simulink model "Robot_Protected_Model"  (Simulink 8.0)
settings: Solver=ode45  StartTime=0.0  StopTime=simtime  RelTol=1e-3
values from neighbouring files (symbols this model uses):
  de = 30*pi/180    (= 0.523598775598)    [Robot_Feedback_Master.m]
  de0 = 0    [Robot_Feedback_Master.m]
  F = [mu1, 0; 0, mu2]    [Robot_Feedback_Master.m]
  g = 9.81    [Robot_Feedback_Master.m]
  Gamma1 = 0.0*diag([1, 1, 1, 1, 1, 1, 1, 1, 1], 0)    [Robot_Feedback_Master.m]
  I1 = 0.12    [Robot_Feedback_Master.m]
  Ie = 0.25    [Robot_Feedback_Master.m]
  Ie0 = 0.12    [Robot_Feedback_Master.m]
  initial_pos = 1*[-3; -3]    [Robot_Feedback_Master.m]
  initial_theta = 0*theta'    [Robot_Feedback_Master.m]
  initial_vel = 1*[-6; 6]    [Robot_Feedback_Master.m]
  KD = 100 * eye(2, 2)    [Robot_Feedback_Master.m]
  L1 = 1    [Robot_Feedback_Master.m]
  lambda = 0    [Robot_Feedback_Master.m]
  Lambda = 10 * eye(2, 2)    [Robot_Feedback_Master.m]
  lambdaf = 100    [Robot_Feedback_Master.m]
  Lc1 = 0.5    [Robot_Feedback_Master.m]
  Lce = 0.6    [Robot_Feedback_Master.m]
  Lce0 = 0.5    [Robot_Feedback_Master.m]
  M1 = 1    [Robot_Feedback_Master.m]
  Me = 5    [Robot_Feedback_Master.m]
  Me0 = 1    [Robot_Feedback_Master.m]
  R = 0 * eye(2, 2)    [Robot_Feedback_Master.m]
  tau1lim = 500    [Robot_Feedback_Master.m]
  tau2lim = 250    [Robot_Feedback_Master.m]
  thetaeps = 10    [Robot_Feedback_Master.m]
  thetamax = 40    [Robot_Feedback_Master.m]
undefined symbols (not defined in the file or in its folder): Gamma
libraries: dspmtrx3 x1
settings Model: Creator=Travis  LastModifiedBy=Dan
settings DataIOCC: SignalLoggingSaveFormat=ModelDataLogs
settings DebuggingCC: FcnCallInpInsideContextMsg=UseLocalSettings
settings GRTTargetCC: CombineOutputUpdateFcns=off  GRTInterface=on

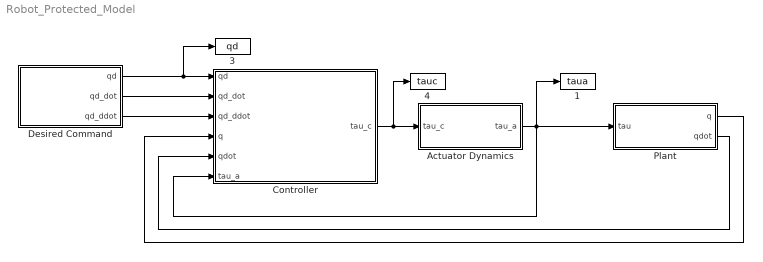
== system Robot_Protected_Model ==
  1 : ToWorkspace  VariableName=taua  SampleTime=-1  SaveFormat=Structure With Time
  3 : ToWorkspace  VariableName=qd  SampleTime=-1  SaveFormat=Structure With Time
  4 : ToWorkspace  VariableName=tauc  SampleTime=-1  SaveFormat=Structure With Time
  Actuator Dynamics : Subsystem
  Controller : Subsystem
  Desired Command : Subsystem
  Plant : Subsystem
  wires:
  Plant/2(qdot) -> Controller/5(qdot)
  Plant/1(q) -> Controller/4(q)
  Controller/1(tau_c) -> 4/1, Actuator Dynamics/1(tau_c)
  Desired Command/1(qd) -> Controller/1(qd), 3/1
  Actuator Dynamics/1(tau_a) -> Controller/6(tau_a), Plant/1(tau), 1/1
  Desired Command/2(qd_dot) -> Controller/2(qd_dot)
  Desired Command/3(qd_ddot) -> Controller/3(qd_ddot)

== system Robot_Protected_Model/Actuator Dynamics ==
  tau_c : Inport
  Demux : Demux  Outputs=2
  Mux : Mux  Inputs=2
  Saturation : Saturate  UpperLimit=tau1lim  LowerLimit=-tau1lim  ZeroCross=off
  Saturation1 : Saturate  UpperLimit=tau2lim  LowerLimit=-tau2lim  ZeroCross=off
  tau_a : Outport
  wires:
  Demux/1 -> Saturation/1
  Saturation/1 -> Mux/1
  Demux/2 -> Saturation1/1
  Saturation1/1 -> Mux/2
  Mux/1 -> tau_a/1
  tau_c/1 -> Demux/1

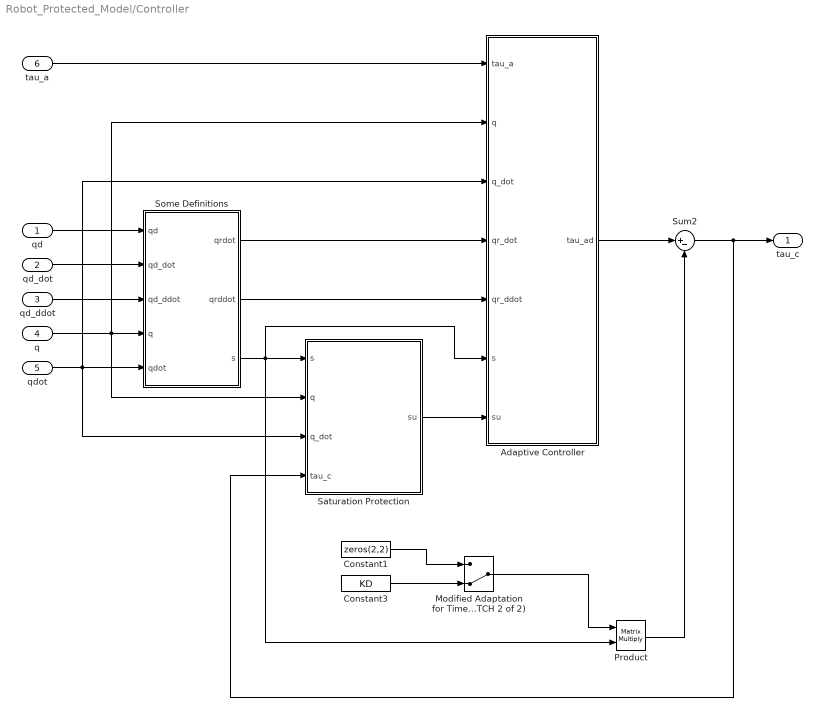
== system Robot_Protected_Model/Controller ==
  qd : Inport
  qd_dot : Inport  Port=2
  qd_ddot : Inport  Port=3
  q : Inport  Port=4
  qdot : Inport  Port=5
  tau_a : Inport  Port=6
  Adaptive Controller : Subsystem
  Constant1 : Constant  Value=zeros(2,2)
  Constant3 : Constant  Value=KD
  Modified Adaptation for Time Varying KD (SWITCH 2 of 2) : ManualSwitch  CurrentSetting=0
  Product : Product  Multiplication=Matrix(*)  RndMeth=Zero
  Saturation Protection : Subsystem
  Some Definitions : Subsystem
  Sum2 : Sum  Inputs=|+-
  tau_c : Outport
  wires:
  Adaptive Controller/1(tau_ad) -> Sum2/1
  Product/1 -> Sum2/2
  Sum2/1 -> tau_c/1, Saturation Protection/4(tau_c)
  q/1 -> Saturation Protection/2(q), Some Definitions/4(q), Adaptive Controller/2(q)
  qdot/1 -> Adaptive Controller/3(q_dot), Saturation Protection/3(q_dot), Some Definitions/5(qdot)
  Some Definitions/1(qrdot) -> Adaptive Controller/4(qr_dot)
  Some Definitions/2(qrddot) -> Adaptive Controller/5(qr_ddot)
  qd_ddot/1 -> Some Definitions/3(qd_ddot)
  qd_dot/1 -> Some Definitions/2(qd_dot)
  qd/1 -> Some Definitions/1(qd)
  Saturation Protection/1(su) -> Adaptive Controller/7(su)
  Some Definitions/3(s) -> Product/2, Adaptive Controller/6(s), Saturation Protection/1(s)
  Constant3/1 -> Modified Adaptation for Time Varying KD (SWITCH 2 of 2)/2
  Constant1/1 -> Modified Adaptation for Time Varying KD (SWITCH 2 of 2)/1
  Modified Adaptation for Time Varying KD (SWITCH 2 of 2)/1 -> Product/1
  tau_a/1 -> Adaptive Controller/1(tau_a)

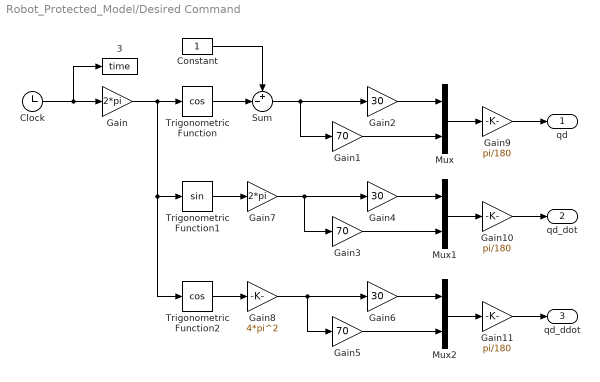
== system Robot_Protected_Model/Desired Command ==
  3 : ToWorkspace  VariableName=time  SampleTime=-1
  Clock : Clock
  Constant : Constant
  Gain : Gain  Gain=2*pi
  Gain1 : Gain  Gain=70
  Gain10 : Gain  Gain=pi/180
  Gain11 : Gain  Gain=pi/180
  Gain2 : Gain  Gain=30
  Gain3 : Gain  Gain=70
  Gain4 : Gain  Gain=30
  Gain5 : Gain  Gain=70
  Gain6 : Gain  Gain=30
  Gain7 : Gain  Gain=2*pi
  Gain8 : Gain  Gain=4*pi^2
  Gain9 : Gain  Gain=pi/180
  Mux : Mux  Inputs=2
  Mux1 : Mux  Inputs=2
  Mux2 : Mux  Inputs=2
  Sum : Sum  Inputs=+-|
  Trigonometric Function : Trigonometry  Operator=cos
  Trigonometric Function1 : Trigonometry
  Trigonometric Function2 : Trigonometry  Operator=cos
  qd : Outport
  qd_dot : Outport  Port=2
  qd_ddot : Outport  Port=3
  wires:
  Clock/1 -> Gain/1, 3/1
  Gain/1 -> Trigonometric Function/1, Trigonometric Function1/1, Trigonometric Function2/1
  Sum/1 -> Gain2/1, Gain1/1
  Gain1/1 -> Mux/2
  Trigonometric Function1/1 -> Gain7/1
  Trigonometric Function2/1 -> Gain8/1
  Mux/1 -> Gain9/1
  Gain2/1 -> Mux/1
  Gain7/1 -> Gain4/1, Gain3/1
  Gain3/1 -> Mux1/2
  Gain4/1 -> Mux1/1
  Gain8/1 -> Gain5/1, Gain6/1
  Gain5/1 -> Mux2/2
  Mux2/1 -> Gain11/1
  Gain6/1 -> Mux2/1
  Mux1/1 -> Gain10/1
  Constant/1 -> Sum/1
  Trigonometric Function/1 -> Sum/2
  Gain9/1 -> qd/1
  Gain10/1 -> qd_dot/1
  Gain11/1 -> qd_ddot/1

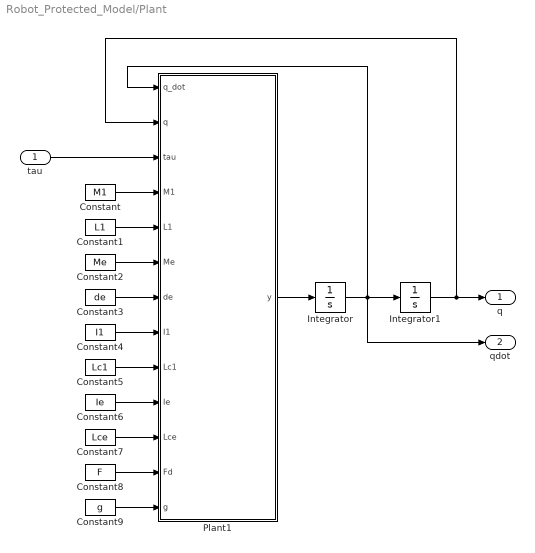
== system Robot_Protected_Model/Plant ==
  tau : Inport
  Constant : Constant  Value=M1
  Constant1 : Constant  Value=L1
  Constant2 : Constant  Value=Me
  Constant3 : Constant  Value=de
  Constant4 : Constant  Value=I1
  Constant5 : Constant  Value=Lc1
  Constant6 : Constant  Value=Ie
  Constant7 : Constant  Value=Lce
  Constant8 : Constant  Value=F
  Constant9 : Constant  Value=g
  Integrator : Integrator  InitialCondition=initial_vel
  Integrator1 : Integrator  InitialCondition=initial_pos
  Plant1 : MATLAB Function  TreatAsAtomicUnit=on
  q : Outport
  qdot : Outport  Port=2
  wires:
  Plant1/1(y) -> Integrator/1
  Integrator/1 -> qdot/1, Plant1/1(q_dot), Integrator1/1
  Constant/1 -> Plant1/4(M1)
  Constant1/1 -> Plant1/5(L1)
  Constant2/1 -> Plant1/6(Me)
  Constant3/1 -> Plant1/7(de)
  Constant5/1 -> Plant1/9(Lc1)
  Constant4/1 -> Plant1/8(I1)
  Constant6/1 -> Plant1/10(Ie)
  Constant7/1 -> Plant1/11(Lce)
  tau/1 -> Plant1/3(tau)
  Integrator1/1 -> Plant1/2(q), q/1
  Constant8/1 -> Plant1/12(Fd)
  Constant9/1 -> Plant1/13(g)

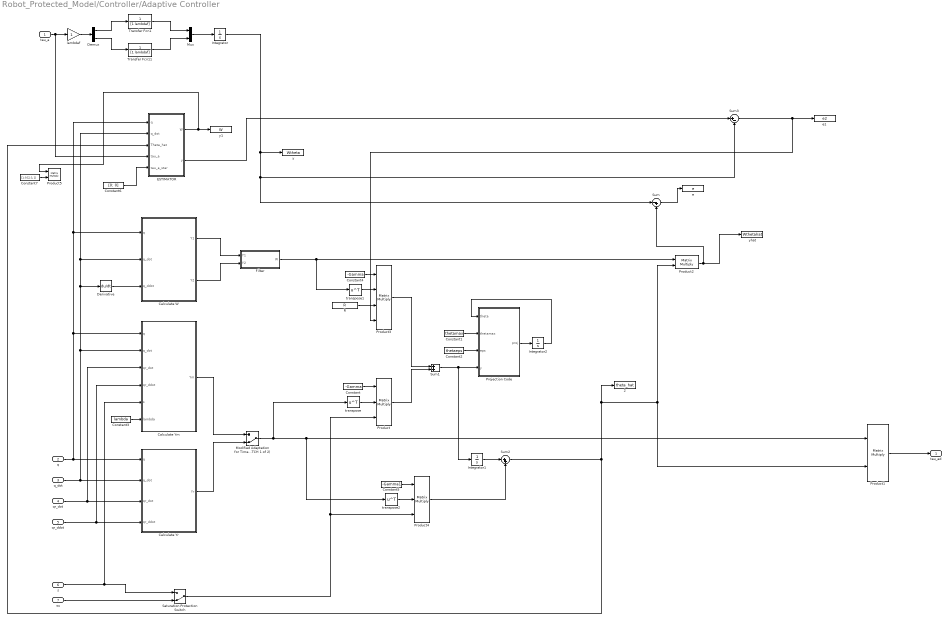
== system Robot_Protected_Model/Controller/Adaptive Controller ==
  tau_a : Inport
  q : Inport  Port=2
  q_dot : Inport  Port=3
  qr_dot : Inport  Port=4
  qr_ddot : Inport  Port=5
  s : Inport  Port=6
  su : Inport  Port=7
  2 : ToWorkspace  VariableName=theta_hat  SampleTime=-1  SaveFormat=Structure With Time
  Calculate W : MATLAB Function  TreatAsAtomicUnit=on
  Calculate Ym : MATLAB Function  TreatAsAtomicUnit=on
  Calculate Yr : MATLAB Function  TreatAsAtomicUnit=on
  Constant : Constant  Value=-Gamma
  Constant1 : Constant  Value=thetamax
  Constant2 : Constant  Value=thetaeps
  Constant3 : Constant  Value=lambda
  Constant4 : Constant  Value=-Gamma
  Constant5 : Constant  Value=-Gamma1
  Constant6 : Constant  Value=[0; 0]
  Constant7 : Constant  Value=[1; 0.12; 1; 1]
  Demux : Demux  Outputs=2
  Derivative : Derivative
  ESTIMATOR : Subsystem
  Filter : Subsystem
  Integrator : Integrator  InitialCondition=[0; 0]
  Integrator1 : Integrator  InitialCondition=initial_theta
  Integrator2 : Integrator  InitialCondition=initial_theta
  Modified Adaptation for Time Varying KD (SWITCH 1 of 2) : ManualSwitch  CurrentSetting=0
  Mux : Mux  Inputs=2
  Product : Product  Inputs=3  Multiplication=Matrix(*)  RndMeth=Zero
  Product1 : Product  Multiplication=Matrix(*)  RndMeth=Zero
  Product2 : Product  Multiplication=Matrix(*)  RndMeth=Zero
  Product3 : Product  Inputs=4  Multiplication=Matrix(*)  RndMeth=Zero
  Product4 : Product  Inputs=3  Multiplication=Matrix(*)  RndMeth=Zero
  Product5 : Product  Multiplication=Matrix(*)  RndMeth=Zero
  Projection Code : Subsystem
  R : Constant  Value=R
  Saturation Protection Switch : ManualSwitch  CurrentSetting=0
  Sum : Sum  Inputs=|-+
  Sum1 : Sum
  Sum2 : Sum  Inputs=|++
  Sum3 : Sum  Inputs=|+-
  Transfer Fcn1 : TransferFcn  Denominator=[1 lambdaf]
  Transfer Fcn11 : TransferFcn  Denominator=[1 lambdaf]
  e : ToWorkspace  VariableName=e  SampleTime=-1  SaveFormat=Structure With Time
  e1 : ToWorkspace  VariableName=e2  SampleTime=-1  SaveFormat=Structure With Time
  lambdaf : Gain
  transpose : Math  Operator=transpose  SaturateOnIntegerOverflow=on
  transpose1 : Math  Operator=transpose  SaturateOnIntegerOverflow=on
  transpose2 : Math  Operator=transpose  SaturateOnIntegerOverflow=on
  y : ToWorkspace  VariableName=Wtheta  SampleTime=-1  SaveFormat=Structure With Time
  y1 : ToWorkspace  VariableName=W  SampleTime=-1  SaveFormat=Structure With Time
  yhat : ToWorkspace  VariableName=Wthetahat  SampleTime=-1  SaveFormat=Structure With Time
  tau_ad : Outport
  wires:
  Constant/1 -> Product/1
  transpose/1 -> Product/2
  Product1/1 -> tau_ad/1
  q/1 -> Calculate Yr/1(q), Calculate Ym/1(q), ESTIMATOR/1(q), Calculate W/1(q)
  qr_ddot/1 -> Calculate Ym/4(qr_ddot), Calculate Yr/4(qr_ddot)
  qr_dot/1 -> Calculate Ym/3(qr_dot), Calculate Yr/3(qr_dot)
  q_dot/1 -> Derivative/1, ESTIMATOR/2(q_dot), Calculate W/2(q_dot), Calculate Ym/2(q_dot), Calculate Yr/2(q_dot)
  s/1 -> Calculate Ym/5(s), Saturation Protection Switch/1
  su/1 -> Saturation Protection Switch/2
  Saturation Protection Switch/1 -> Product4/3, Product/3
  Constant3/1 -> Calculate Ym/6(lambda)
  Modified Adaptation for Time Varying KD (SWITCH 1 of 2)/1 -> transpose/1, transpose2/1, Product1/1
  Calculate Ym/1(Ym) -> Modified Adaptation for Time Varying KD (SWITCH 1 of 2)/1
  Calculate Yr/1(Yr) -> Modified Adaptation for Time Varying KD (SWITCH 1 of 2)/2
  Derivative/1 -> Calculate W/3(q_ddot)
  Calculate W/1(Y1) -> Filter/1(Y1)
  Calculate W/2(Y2) -> Filter/2(Y2)
  Demux/1 -> Transfer Fcn1/1
  Demux/2 -> Transfer Fcn11/1
  tau_a/1 -> ESTIMATOR/4(tau_a), lambdaf/1
  Transfer Fcn1/1 -> Mux/1
  Transfer Fcn11/1 -> Mux/2
  Mux/1 -> Integrator/1
  Filter/1(W) -> transpose1/1, Product2/1
  Integrator/1 -> Sum3/2, Sum/1, y/1
  Product2/1 -> yhat/1, Sum/2
  Sum/1 -> e/1
  Projection Code/1(proj) -> Integrator2/1
  Constant1/1 -> Projection Code/2(thetamax)
  Constant2/1 -> Projection Code/3(eps)
  Sum2/1 -> 2/1, Product1/2, Product2/2, ESTIMATOR/3(Theta_hat)
  Constant4/1 -> Product3/1
  transpose1/1 -> Product3/2
  R/1 -> Product3/3
  Product3/1 -> Sum1/1
  Product/1 -> Sum1/2
  Sum1/1 -> Integrator1/1, Projection Code/4(y)
  lambdaf/1 -> Demux/1
  Integrator2/1 -> Projection Code/1(theta)
  Constant5/1 -> Product4/1
  transpose2/1 -> Product4/2
  Product4/1 -> Sum2/2
  ESTIMATOR/1(W) -> Product5/1, y1/1
  Integrator1/1 -> Sum2/1
  Constant7/1 -> Product5/2
  ESTIMATOR/2(y) -> Sum3/1
  Sum3/1 -> Product3/4, e1/1
  Constant6/1 -> ESTIMATOR/5(tau_a_star)

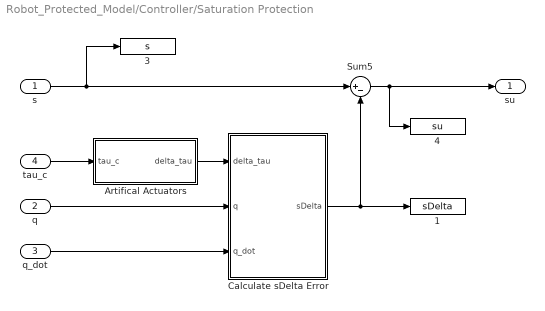
== system Robot_Protected_Model/Controller/Saturation Protection ==
  s : Inport
  q : Inport  Port=2
  q_dot : Inport  Port=3
  tau_c : Inport  Port=4
  1 : ToWorkspace  VariableName=sDelta  SampleTime=-1  SaveFormat=Structure With Time
  3 : ToWorkspace  VariableName=s  SampleTime=-1  SaveFormat=Structure With Time
  4 : ToWorkspace  VariableName=su  SampleTime=-1  SaveFormat=Structure With Time
  Artifical Actuators : Subsystem
  "Calculate sDelta Error " : Subsystem
  Sum5 : Sum  Inputs=|+-
  su : Outport
  wires:
  q/1 -> "Calculate sDelta Error "/2(q)
  q_dot/1 -> "Calculate sDelta Error "/3(q_dot)
  Artifical Actuators/1(delta_tau) -> "Calculate sDelta Error "/1(delta_tau)
  s/1 -> 3/1, Sum5/1
  Sum5/1 -> su/1, 4/1
  "Calculate sDelta Error "/1(sDelta) -> 1/1, Sum5/2
  tau_c/1 -> Artifical Actuators/1(tau_c)

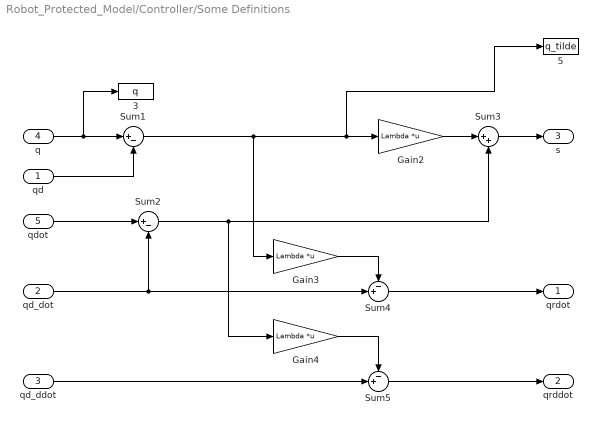
== system Robot_Protected_Model/Controller/Some Definitions ==
  qd : Inport
  qd_dot : Inport  Port=2
  qd_ddot : Inport  Port=3
  q : Inport  Port=4
  qdot : Inport  Port=5
  3 : ToWorkspace  VariableName=q  SampleTime=-1  SaveFormat=Structure With Time
  5 : ToWorkspace  VariableName=q_tilde  SampleTime=-1  SaveFormat=Structure With Time
  Gain2 : Gain  Gain=Lambda  Multiplication=Matrix(K*u)
  Gain3 : Gain  Gain=Lambda  Multiplication=Matrix(K*u)
  Gain4 : Gain  Gain=Lambda  Multiplication=Matrix(K*u)
  Sum1 : Sum  Inputs=|+-
  Sum2 : Sum  Inputs=|+-
  Sum3 : Sum  Inputs=|++
  Sum4 : Sum  Inputs=-+|
  Sum5 : Sum  Inputs=-+|
  qrdot : Outport
  qrddot : Outport  Port=2
  s : Outport  Port=3
  wires:
  qd/1 -> Sum1/2
  qd_dot/1 -> Sum2/2, Sum4/2
  q/1 -> 3/1, Sum1/1
  Sum1/1 -> Gain3/1, 5/1, Gain2/1
  qdot/1 -> Sum2/1
  Sum2/1 -> Sum3/2, Gain4/1
  Gain2/1 -> Sum3/1
  Sum3/1 -> s/1
  Sum4/1 -> qrdot/1
  Sum5/1 -> qrddot/1
  Gain3/1 -> Sum4/1
  Gain4/1 -> Sum5/1
  qd_ddot/1 -> Sum5/2

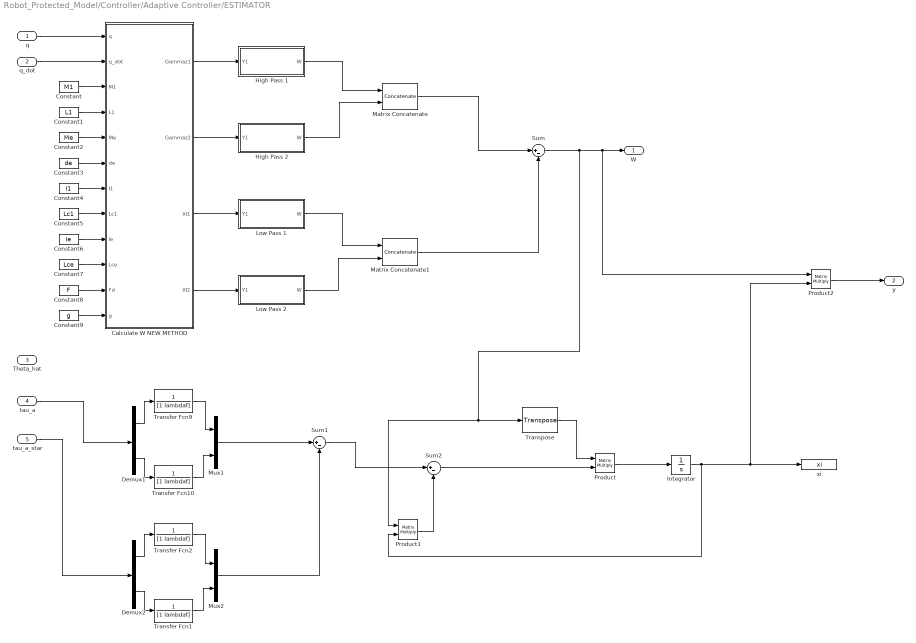
== system Robot_Protected_Model/Controller/Adaptive Controller/ESTIMATOR ==
  q : Inport
  q_dot : Inport  Port=2
  Theta_hat : Inport  Port=3
  tau_a : Inport  Port=4
  tau_a_star : Inport  Port=5
  Calculate W NEW METHOD : MATLAB Function  TreatAsAtomicUnit=on
  Constant : Constant  Value=M1
  Constant1 : Constant  Value=L1
  Constant2 : Constant  Value=Me
  Constant3 : Constant  Value=de
  Constant4 : Constant  Value=I1
  Constant5 : Constant  Value=Lc1
  Constant6 : Constant  Value=Ie
  Constant7 : Constant  Value=Lce
  Constant8 : Constant  Value=F
  Constant9 : Constant  Value=g
  Demux1 : Demux  Outputs=2
  Demux2 : Demux  Outputs=2
  High Pass 1 : Subsystem
  High Pass 2 : Subsystem
  Integrator : Integrator  InitialCondition=[0; 0; 0; 0]
  Low Pass 1 : Subsystem
  Low Pass 2 : Subsystem
  Matrix Concatenate : Concatenate  Mode=Multidimensional array
  Matrix Concatenate1 : Concatenate  Mode=Multidimensional array
  Mux1 : Mux  Inputs=2
  Mux2 : Mux  Inputs=2
  Product : Product  Multiplication=Matrix(*)  RndMeth=Zero
  Product1 : Product  Multiplication=Matrix(*)  RndMeth=Zero
  Product2 : Product  Multiplication=Matrix(*)  RndMeth=Zero
  Sum : Sum  Inputs=|+-
  Sum1 : Sum  Inputs=|+-
  Sum2 : Sum  Inputs=|+-
  Transfer Fcn{1..2,9..10} (4 alike) : TransferFcn  Denominator=[1 lambdaf]
  Transpose : dspmtrx3/Transpose  Hermitian=off  overflowFlag=off
  xi : ToWorkspace  VariableName=xi  SampleTime=-1  SaveFormat=Structure With Time
  W : Outport
  y : Outport  Port=2
  wires:
  Constant/1 -> Calculate W NEW METHOD/3(M1)
  Constant1/1 -> Calculate W NEW METHOD/4(L1)
  Constant2/1 -> Calculate W NEW METHOD/5(Me)
  Constant3/1 -> Calculate W NEW METHOD/6(de)
  Constant4/1 -> Calculate W NEW METHOD/7(I1)
  Constant5/1 -> Calculate W NEW METHOD/8(Lc1)
  Constant6/1 -> Calculate W NEW METHOD/9(Ie)
  Constant7/1 -> Calculate W NEW METHOD/10(Lce)
  Constant8/1 -> Calculate W NEW METHOD/11(Fd)
  Constant9/1 -> Calculate W NEW METHOD/12(g)
  q/1 -> Calculate W NEW METHOD/1(q)
  q_dot/1 -> Calculate W NEW METHOD/2(q_dot)
  Calculate W NEW METHOD/3(XI1) -> Low Pass 1/1(Y1)
  Calculate W NEW METHOD/4(XI2) -> Low Pass 2/1(Y1)
  Calculate W NEW METHOD/2(Gammaz2) -> High Pass 2/1(Y1)
  Calculate W NEW METHOD/1(Gammaz1) -> High Pass 1/1(Y1)
  High Pass 1/1(W) -> Matrix Concatenate/1
  High Pass 2/1(W) -> Matrix Concatenate/2
  Low Pass 1/1(W) -> Matrix Concatenate1/1
  Low Pass 2/1(W) -> Matrix Concatenate1/2
  Matrix Concatenate/1 -> Sum/1
  Matrix Concatenate1/1 -> Sum/2
  Sum/1 -> Product1/1, Transpose/1, Product2/1, W/1
  Demux1/1 -> Transfer Fcn9/1
  Transfer Fcn9/1 -> Mux1/1
  Demux1/2 -> Transfer Fcn10/1
  Transfer Fcn10/1 -> Mux1/2
  Demux2/1 -> Transfer Fcn2/1
  Transfer Fcn2/1 -> Mux2/1
  Demux2/2 -> Transfer Fcn1/1
  Transfer Fcn1/1 -> Mux2/2
  tau_a/1 -> Demux1/1
  tau_a_star/1 -> Demux2/1
  Mux1/1 -> Sum1/1
  Mux2/1 -> Sum1/2
  Transpose/1 -> Product/1
  Sum2/1 -> Product/2
  Product/1 -> Integrator/1
  Sum1/1 -> Sum2/1
  Product1/1 -> Sum2/2
  Integrator/1 -> Product1/2, Product2/2, xi/1
  Product2/1 -> y/1

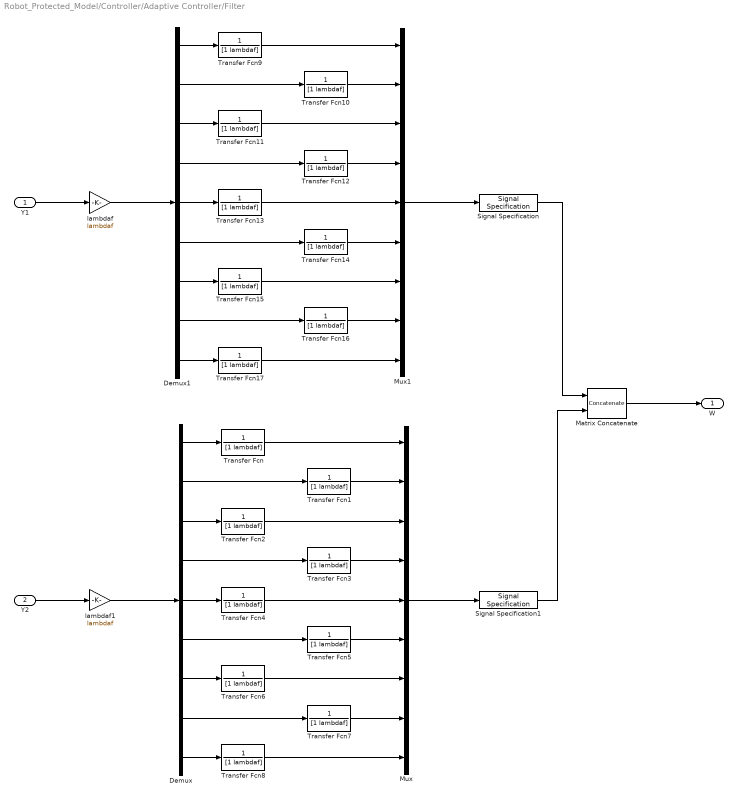
== system Robot_Protected_Model/Controller/Adaptive Controller/Filter ==
  Y1 : Inport
  Y2 : Inport  Port=2
  Demux : Demux  Outputs=9
  Demux1 : Demux  Outputs=9
  Matrix Concatenate : Concatenate  Mode=Multidimensional array
  Mux : Mux  Inputs=9
  Mux1 : Mux  Inputs=9
  Signal Specification : SignalSpecification  Dimensions=[1,9]
  Signal Specification1 : SignalSpecification  Dimensions=[1,9]
  Transfer Fcn{,1..17} (18 alike) : TransferFcn  Denominator=[1 lambdaf]
  lambdaf : Gain  Gain=lambdaf
  lambdaf1 : Gain  Gain=lambdaf
  W : Outport
  wires:
  Demux/1 -> Transfer Fcn/1
  Transfer Fcn/1 -> Mux/1
  Demux/2 -> Transfer Fcn1/1
  Transfer Fcn1/1 -> Mux/2
  Transfer Fcn2/1 -> Mux/3
  Demux/4 -> Transfer Fcn3/1
  Transfer Fcn4/1 -> Mux/5
  Demux/6 -> Transfer Fcn5/1
  Transfer Fcn6/1 -> Mux/7
  Demux/8 -> Transfer Fcn7/1
  Demux/3 -> Transfer Fcn2/1
  Transfer Fcn3/1 -> Mux/4
  Demux/5 -> Transfer Fcn4/1
  Transfer Fcn5/1 -> Mux/6
  Demux/7 -> Transfer Fcn6/1
  Transfer Fcn7/1 -> Mux/8
  Demux/9 -> Transfer Fcn8/1
  Transfer Fcn8/1 -> Mux/9
  Demux1/1 -> Transfer Fcn9/1
  Transfer Fcn9/1 -> Mux1/1
  Demux1/2 -> Transfer Fcn10/1
  Transfer Fcn10/1 -> Mux1/2
  Transfer Fcn11/1 -> Mux1/3
  Demux1/4 -> Transfer Fcn12/1
  Transfer Fcn13/1 -> Mux1/5
  Demux1/6 -> Transfer Fcn14/1
  Transfer Fcn15/1 -> Mux1/7
  Demux1/8 -> Transfer Fcn16/1
  Demux1/3 -> Transfer Fcn11/1
  Transfer Fcn12/1 -> Mux1/4
  Demux1/5 -> Transfer Fcn13/1
  Transfer Fcn14/1 -> Mux1/6
  Demux1/7 -> Transfer Fcn15/1
  Transfer Fcn16/1 -> Mux1/8
  Demux1/9 -> Transfer Fcn17/1
  Transfer Fcn17/1 -> Mux1/9
  Y1/1 -> lambdaf/1
  Y2/1 -> lambdaf1/1
  Mux1/1 -> Signal Specification/1
  Mux/1 -> Signal Specification1/1
  Signal Specification/1 -> Matrix Concatenate/1
  Signal Specification1/1 -> Matrix Concatenate/2
  Matrix Concatenate/1 -> W/1
  lambdaf1/1 -> Demux/1
  lambdaf/1 -> Demux1/1

== system Robot_Protected_Model/Controller/Adaptive Controller/Projection Code ==
  note: This block is the projection operator. See notes.
  theta : Inport
  thetamax : Inport  Port=2
  eps : Inport  Port=3
  y : Inport  Port=4
  Projection : MATLAB Function  TreatAsAtomicUnit=on
  proj : Outport
  wires:
  Projection/1(proj) -> proj/1
  theta/1 -> Projection/1(theta)
  thetamax/1 -> Projection/2(thetamax)
  eps/1 -> Projection/3(eps)
  y/1 -> Projection/4(y)

== system Robot_Protected_Model/Controller/Saturation Protection/Artifical Actuators ==
  tau_c : Inport
  Demux : Demux  Outputs=2
  Mux : Mux  Inputs=2
  Saturation : Saturate  UpperLimit=tau1lim  LowerLimit=-tau1lim  ZeroCross=off
  Saturation1 : Saturate  UpperLimit=tau2lim  LowerLimit=-tau2lim  ZeroCross=off
  Sum : Sum  Inputs=|-+
  delta_tau : Outport
  wires:
  Demux/1 -> Saturation/1
  Saturation/1 -> Mux/1
  Demux/2 -> Saturation1/1
  Saturation1/1 -> Mux/2
  tau_c/1 -> Sum/1, Demux/1
  Mux/1 -> Sum/2
  Sum/1 -> delta_tau/1

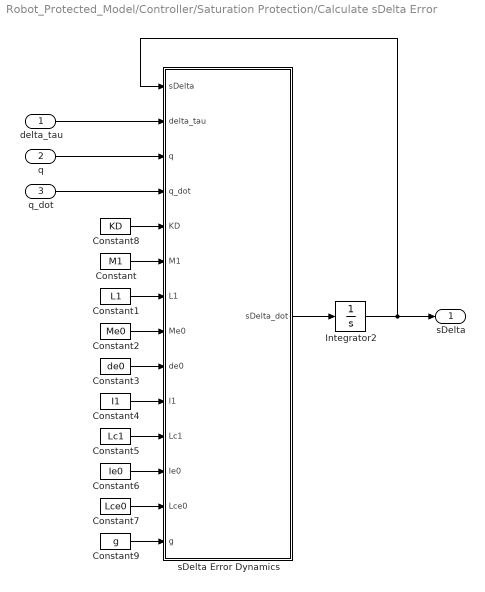
== system Robot_Protected_Model/Controller/Saturation Protection/Calculate sDelta Error  ==
  delta_tau : Inport
  q : Inport  Port=2
  q_dot : Inport  Port=3
  Constant : Constant  Value=M1
  Constant1 : Constant  Value=L1
  Constant2 : Constant  Value=Me0
  Constant3 : Constant  Value=de0
  Constant4 : Constant  Value=I1
  Constant5 : Constant  Value=Lc1
  Constant6 : Constant  Value=Ie0
  Constant7 : Constant  Value=Lce0
  Constant8 : Constant  Value=KD
  Constant9 : Constant  Value=g
  Integrator2 : Integrator  InitialCondition=[0;0];
  sDelta Error Dynamics : MATLAB Function  TreatAsAtomicUnit=on
  sDelta : Outport
  wires:
  delta_tau/1 -> sDelta Error Dynamics/2(delta_tau)
  sDelta Error Dynamics/1(sDelta_dot) -> Integrator2/1
  Integrator2/1 -> sDelta Error Dynamics/1(sDelta), sDelta/1
  Constant/1 -> sDelta Error Dynamics/6(M1)
  Constant1/1 -> sDelta Error Dynamics/7(L1)
  Constant2/1 -> sDelta Error Dynamics/8(Me0)
  Constant3/1 -> sDelta Error Dynamics/9(de0)
  Constant4/1 -> sDelta Error Dynamics/10(I1)
  Constant5/1 -> sDelta Error Dynamics/11(Lc1)
  Constant6/1 -> sDelta Error Dynamics/12(Ie0)
  Constant7/1 -> sDelta Error Dynamics/13(Lce0)
  q/1 -> sDelta Error Dynamics/3(q)
  q_dot/1 -> sDelta Error Dynamics/4(q_dot)
  Constant8/1 -> sDelta Error Dynamics/5(KD)
  Constant9/1 -> sDelta Error Dynamics/14(g)

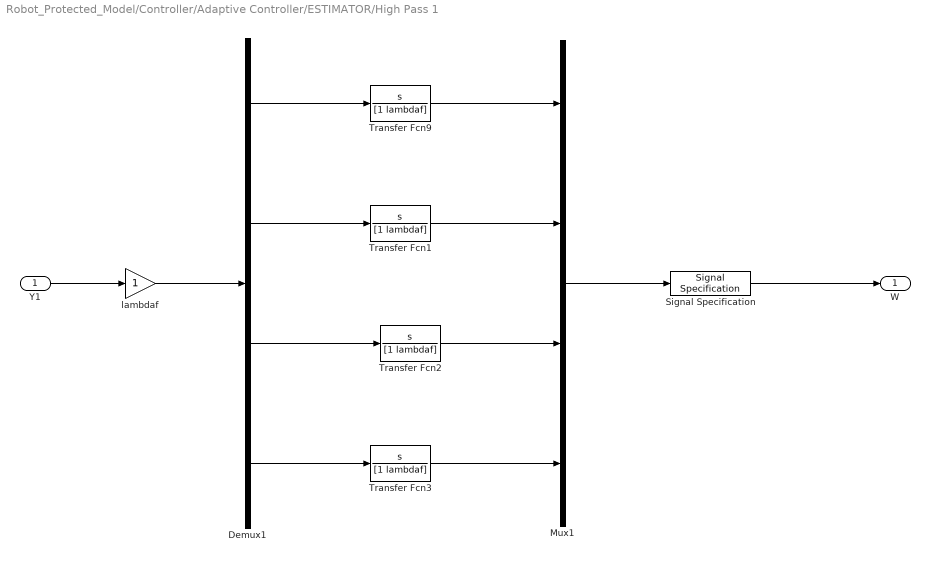
== system Robot_Protected_Model/Controller/Adaptive Controller/ESTIMATOR/High Pass 1 ==
  Y1 : Inport
  Demux1 : Demux
  Mux1 : Mux
  Signal Specification : SignalSpecification  Dimensions=[1,4]
  Transfer Fcn{1..3,9} (4 alike) : TransferFcn  Numerator=[1 0]  Denominator=[1 lambdaf]
  lambdaf : Gain
  W : Outport
  wires:
  Demux1/1 -> Transfer Fcn9/1
  Transfer Fcn9/1 -> Mux1/1
  Demux1/2 -> Transfer Fcn1/1
  Transfer Fcn1/1 -> Mux1/2
  Transfer Fcn2/1 -> Mux1/3
  Demux1/4 -> Transfer Fcn3/1
  Demux1/3 -> Transfer Fcn2/1
  Transfer Fcn3/1 -> Mux1/4
  Y1/1 -> lambdaf/1
  Mux1/1 -> Signal Specification/1
  lambdaf/1 -> Demux1/1
  Signal Specification/1 -> W/1

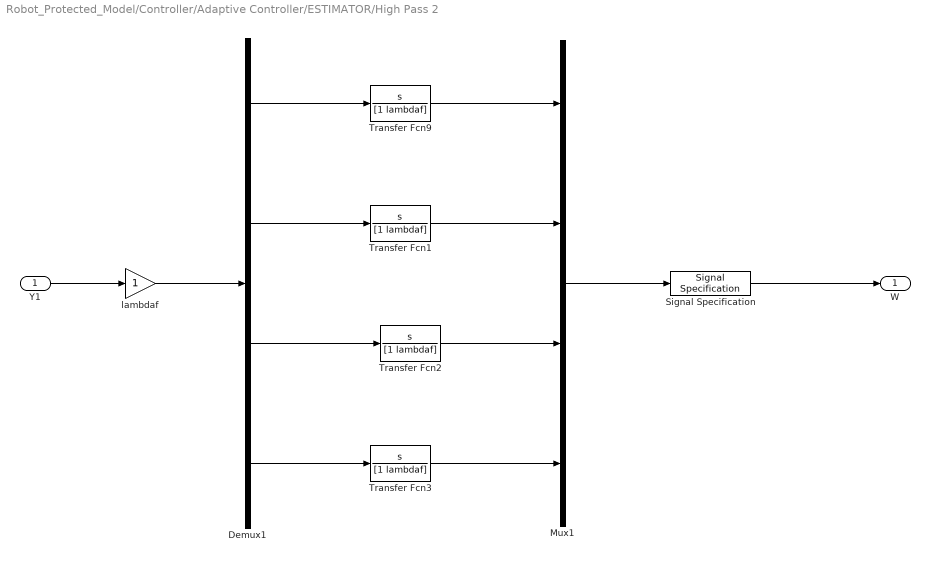
== system Robot_Protected_Model/Controller/Adaptive Controller/ESTIMATOR/High Pass 2 ==
  Y1 : Inport
  Demux1 : Demux
  Mux1 : Mux
  Signal Specification : SignalSpecification  Dimensions=[1,4]
  Transfer Fcn{1..3,9} (4 alike) : TransferFcn  Numerator=[1 0]  Denominator=[1 lambdaf]
  lambdaf : Gain
  W : Outport
  wires:
  Demux1/1 -> Transfer Fcn9/1
  Transfer Fcn9/1 -> Mux1/1
  Demux1/2 -> Transfer Fcn1/1
  Transfer Fcn1/1 -> Mux1/2
  Transfer Fcn2/1 -> Mux1/3
  Demux1/4 -> Transfer Fcn3/1
  Demux1/3 -> Transfer Fcn2/1
  Transfer Fcn3/1 -> Mux1/4
  Y1/1 -> lambdaf/1
  Mux1/1 -> Signal Specification/1
  lambdaf/1 -> Demux1/1
  Signal Specification/1 -> W/1

== system Robot_Protected_Model/Controller/Adaptive Controller/ESTIMATOR/Low Pass 1 ==
  Y1 : Inport
  Demux1 : Demux
  Mux1 : Mux
  Signal Specification : SignalSpecification  Dimensions=[1,4]
  Transfer Fcn{9..12} (4 alike) : TransferFcn  Denominator=[1 lambdaf]
  lambdaf : Gain
  W : Outport
  wires:
  Demux1/1 -> Transfer Fcn9/1
  Transfer Fcn9/1 -> Mux1/1
  Demux1/2 -> Transfer Fcn10/1
  Transfer Fcn10/1 -> Mux1/2
  Transfer Fcn11/1 -> Mux1/3
  Demux1/4 -> Transfer Fcn12/1
  Demux1/3 -> Transfer Fcn11/1
  Transfer Fcn12/1 -> Mux1/4
  Y1/1 -> lambdaf/1
  Mux1/1 -> Signal Specification/1
  lambdaf/1 -> Demux1/1
  Signal Specification/1 -> W/1

== system Robot_Protected_Model/Controller/Adaptive Controller/ESTIMATOR/Low Pass 2 ==
  Y1 : Inport
  Demux1 : Demux
  Mux1 : Mux
  Signal Specification : SignalSpecification  Dimensions=[1,4]
  Transfer Fcn{9..12} (4 alike) : TransferFcn  Denominator=[1 lambdaf]
  lambdaf : Gain
  W : Outport
  wires:
  Demux1/1 -> Transfer Fcn9/1
  Transfer Fcn9/1 -> Mux1/1
  Demux1/2 -> Transfer Fcn10/1
  Transfer Fcn10/1 -> Mux1/2
  Transfer Fcn11/1 -> Mux1/3
  Demux1/4 -> Transfer Fcn12/1
  Demux1/3 -> Transfer Fcn11/1
  Transfer Fcn12/1 -> Mux1/4
  Y1/1 -> lambdaf/1
  Mux1/1 -> Signal Specification/1
  lambdaf/1 -> Demux1/1
  Signal Specification/1 -> W/1

== matlab function Controller/Adaptive Controller/Calculate Yr ==
  data: q input double; q_dot input double; qr_dot input double; qr_ddot input double; Yr output double
%%%%%%%%%%%%%%%%%%%%%%%%%%%%%%%%%%%%%%%%%%%%%%%%%%%%%%%%%%%%%%%%%%%%%%%%%%%
% Daniel Wiese
% 2.152
% Robot Manipulator
%--------------------------------------------------------------------------
% Robot
%%%%%%%%%%%%%%%%%%%%%%%%%%%%%%%%%%%%%%%%%%%%%%%%%%%%%%%%%%%%%%%%%%%%%%%%%%%
function Yr=fcn(q,q_dot,qr_dot,qr_ddot)
%#codegen
%Preallocate output
Yr=zeros(2,9);
%Take apart the input
q1=q(1);
q2=q(2);
q_dot1=q_dot(1);
q_dot2=q_dot(2);
qr_dot1=qr_dot(1);
qr_dot2=qr_dot(2);
qr_ddot1=qr_ddot(1);
qr_ddot2=qr_ddot(2);
%Calculate the first row of Y
Yr(1,1)=qr_ddot1;
Yr(1,2)=qr_ddot2;
Yr(1,3)=(2*qr_ddot1+qr_ddot2)*cos(q2)-(q_dot2*qr_dot1+q_dot1*qr_dot2+q_dot2*qr_dot2)*sin(q2);
Yr(1,4)=(2*qr_ddot1+qr_ddot2)*sin(q2)+(q_dot2*qr_dot1+q_dot1*qr_dot2+q_dot2*qr_dot2)*cos(q2);
Yr(1,5)=cos(q1);
Yr(1,6)=cos(q1+q2);
Yr(1,7)=-sin(q1+q2);
Yr(1,8)=q_dot1;
Yr(1,9)=0;
%Calculate the second row of Y
Yr(2,1)=0;
Yr(2,2)=qr_ddot1+qr_ddot2;
Yr(2,3)=qr_ddot1*cos(q2)+q_dot1*qr_dot1*sin(q2);
Yr(2,4)=qr_ddot1*sin(q2)-q_dot1*qr_dot1*cos(q2);
Yr(2,5)=0;
Yr(2,6)=cos(q1+q2);
Yr(2,7)=-sin(q1+q2);
Yr(2,8)=0;
Yr(2,9)=q_dot2;

== matlab function Controller/Saturation Protection/Calculate sDelta Error /sDelta Error Dynamics ==
  data: sDelta input double; sDelta_dot output double; delta_tau input double; q input double; q_dot input double; KD input double; M1 input double; L1 input double; Me0 input double; de0 input double; I1 input double; Lc1 input double; Ie0 input double; Lce0 input double; g input double
%%%%%%%%%%%%%%%%%%%%%%%%%%%%%%%%%%%%%%%%%%%%%%%%%%%%%%%%%%%%%%%%%%%%%%%%%%%
% Daniel Wiese
% 2.152
% Robot Manipulator
%--------------------------------------------------------------------------
% Robot manipulator. See Slotine, Li page 396 for the equations and all of
% the parameter values used.
%%%%%%%%%%%%%%%%%%%%%%%%%%%%%%%%%%%%%%%%%%%%%%%%%%%%%%%%%%%%%%%%%%%%%%%%%%%
function sDelta_dot = fcn(sDelta,delta_tau,q,q_dot,KD,M1,L1,Me0,de0,I1,Lc1,Ie0,Lce0,g)
%#codegen
%Take apart the input
q1=q(1);
q2=q(2);
qdot1=q_dot(1);
qdot2=q_dot(2);
%Define the nominal parameters
theta1=I1+M1*Lc1^2+Ie0+Me0*Lc1^2+Me0*L1^2;
theta2=Ie0+Me0*Lce0^2;
theta3=Me0*L1*Lce0*cos(de0);
theta4=Me0*L1*Lce0*sin(de0);
%Components of the matrix H
H11=theta1+2*theta3*cos(q2)+2*theta4*sin(q2);
H12=theta2+theta3*cos(q2)+theta4*sin(q2);
H21=H12;
H22=theta2;
h=theta3*sin(q2)-theta4*cos(q2);
%The gravity matrix G
G=[(M1*Lc1+Me0*L1)*g*cos(q1)+((Me0*Lce0*g)/cos(de0))*cos(q1+q2+de0);
    ((Me0*Lce0*g)/cos(de0))*cos(q1+q2+de0)];
%Assemble H and C
H=[H11 H12; H21 H22];
C=[-h*qdot2 -h*(qdot1+qdot2); h*qdot1 0];
%Calculate sDelta
sDelta_dot=-H\(C+KD)*sDelta+H\delta_tau;
% sDelta_dot=-10*eye(2,2)*sDelta+0.1*eye(2,2)*delta_tau;

== matlab function Controller/Adaptive Controller/Projection Code/Projection ==
  data: theta input double; thetamax input double; eps input double; proj output double; y input double
%%%%%%%%%%%%%%%%%%%%%%%%%%%%%%%%%%%%%%%%%%%%%%%%%%%%%%%%%%%%%%%%%%%%%%%%%%%
% Daniel Wiese
% Generic Hypersonic Vehicle
% Projection Operator
% 2012-06-05
%--------------------------------------------------------------------------
% This function is the projection algorithm for use in an adaptive control
% law. The inputs are the outer ball radius, and inner radius scaling 
% factor epsilon, which determines the inner radius of the ball. See notes
% for more information.
%%%%%%%%%%%%%%%%%%%%%%%%%%%%%%%%%%%%%%%%%%%%%%%%%%%%%%%%%%%%%%%%%%%%%%%%%%%
function proj=projection(theta,thetamax,eps,y)
%Preallocate
[n,m]=size(theta);
f=zeros(m,1);
gradf=zeros(n,m);
proj=zeros(n,m);
cond=zeros(m,1);
%Projection
for i=1:m
    f(i)=(norm(theta(:,i),2)^2-thetamax(i)^2)/(2*eps(i)*thetamax(i)+eps(i)^2);
    for j=1:n
        gradf(j,i)=(2*theta(j,i))/(2*eps(i)*thetamax(i)+eps(i)^2);
    end
    cond(i)=(f(i)>0 && y(:,i)'*gradf(:,i)>0 );
    if cond(i);
        proj(:,i)=y(:,i)-(gradf(:,i)*gradf(:,i)')/(gradf(:,i)'*gradf(:,i))*y(:,i)*f(i);
    else
        proj(:,i)=y(:,i);
    end
end
%%%%%%%%%%%%%%%%%%%%%%%%%%%%%%%%%%%%%%%%%%%%%%%%%%%%%%%%%%%%%%%%%%%%%%%%%%%

== matlab function Plant/Plant1 ==
  data: q_dot input double; q input double; y output double; tau input double; M1 input double; L1 input double; Me input double; de input double; I1 input double; Lc1 input double; Ie input double; Lce input double; Fd input double; g input double
%%%%%%%%%%%%%%%%%%%%%%%%%%%%%%%%%%%%%%%%%%%%%%%%%%%%%%%%%%%%%%%%%%%%%%%%%%%
% Daniel Wiese
% 2.152
% Robot Manipulator
%--------------------------------------------------------------------------
% Robot manipulator. See Slotine, Li page 396 for the equations and all of
% the parameter values used.
%%%%%%%%%%%%%%%%%%%%%%%%%%%%%%%%%%%%%%%%%%%%%%%%%%%%%%%%%%%%%%%%%%%%%%%%%%%
function y = fcn(q_dot,q,tau,M1,L1,Me,de,I1,Lc1,Ie,Lce,Fd,g)
%#codegen
%Take apart the input
q1=q(1);
q2=q(2);
qdot1=q_dot(1);
qdot2=q_dot(2);
%Define the 'a' parameters
a1=I1+M1*Lc1^2+Ie+Me*Lc1^2+Me*L1^2;
a2=Ie+Me*Lce^2;
a3=Me*L1*Lce*cos(de);
a4=Me*L1*Lce*sin(de);
%Components of the matrix H
H11=a1+2*a3*cos(q2)+2*a4*sin(q2);
H12=a2+a3*cos(q2)+a4*sin(q2);
H21=H12;
H22=a2;
h=a3*sin(q2)-a4*cos(q2);
%The gravity matrix G
G=[(M1*Lc1+Me*L1)*g*cos(q1)+((Me*Lce*g)/cos(de))*cos(q1+q2+de);
    ((Me*Lce*g)/cos(de))*cos(q1+q2+de)];
%Assemble H and C
H=[H11 H12; H21 H22];
C=[-h*qdot2 -h*(qdot1+qdot2); h*qdot1 0];
%Calculate the plant output y=q_ddot
y = -(H\C)*q_dot-(H\G)-(H\Fd)*q_dot+inv(H)*tau;

== matlab function Controller/Adaptive Controller/Calculate Ym ==
  data: q input double; q_dot input double; qr_dot input double; qr_ddot input double; s input double; lambda input double; Ym output double
%%%%%%%%%%%%%%%%%%%%%%%%%%%%%%%%%%%%%%%%%%%%%%%%%%%%%%%%%%%%%%%%%%%%%%%%%%%
% Daniel Wiese
% 2.152
% Robot Manipulator
%--------------------------------------------------------------------------
% Robot
%%%%%%%%%%%%%%%%%%%%%%%%%%%%%%%%%%%%%%%%%%%%%%%%%%%%%%%%%%%%%%%%%%%%%%%%%%%
function Ym=fcn(q,q_dot,qr_dot,qr_ddot,s,lambda)
%#codegen
%Preallocate output
Ym=zeros(2,9);
%Take apart the input
q1=q(1);
q2=q(2);
q_dot1=q_dot(1);
q_dot2=q_dot(2);
qr_dot1=qr_dot(1);
qr_dot2=qr_dot(2);
qr_ddot1=qr_ddot(1);
qr_ddot2=qr_ddot(2);
Ls1=lambda*s(1);
Ls2=lambda*s(2);
qr_ddot1=qr_ddot(1)-Ls1;
qr_ddot2=qr_ddot(2)-Ls2;
%Calculate the first row of Y
Ym(1,1)=qr_ddot1;
Ym(1,2)=qr_ddot2;
Ym(1,3)=(2*qr_ddot1+qr_ddot2)*cos(q2)-(q_dot2*qr_dot1+q_dot1*qr_dot2+q_dot2*qr_dot2)*sin(q2);
Ym(1,4)=(2*qr_ddot1+qr_ddot2)*sin(q2)+(q_dot2*qr_dot1+q_dot1*qr_dot2+q_dot2*qr_dot2)*cos(q2);
Ym(1,5)=cos(q1);
Ym(1,6)=cos(q1+q2);
Ym(1,7)=-sin(q1+q2);
Ym(1,8)=q_dot1;
Ym(1,9)=0;
%Calculate the second row of Y
Ym(2,1)=0;
Ym(2,2)=qr_ddot1+qr_ddot2;
Ym(2,3)=qr_ddot1*cos(q2)+q_dot1*qr_dot1*sin(q2);
Ym(2,4)=qr_ddot1*sin(q2)-q_dot1*qr_dot1*cos(q2);
Ym(2,5)=0;
Ym(2,6)=cos(q1+q2);
Ym(2,7)=-sin(q1+q2);
Ym(2,8)=0;
Ym(2,9)=q_dot2;

== matlab function Controller/Adaptive Controller/ESTIMATOR/Calculate W NEW METHOD ==
  data: q input double; q_dot input double; Gammaz1 output double; Gammaz2 output double; XI1 output double; M1 input double; L1 input double; Me input double; de input double; I1 input double; Lc1 input double; Ie input double; Lce input double; Fd input double; g input double; XI2 output double
%%%%%%%%%%%%%%%%%%%%%%%%%%%%%%%%%%%%%%%%%%%%%%%%%%%%%%%%%%%%%%%%%%%%%%%%%%%
% Daniel Wiese
% 2.152
% Robot Manipulator
%--------------------------------------------------------------------------
% Robot
%%%%%%%%%%%%%%%%%%%%%%%%%%%%%%%%%%%%%%%%%%%%%%%%%%%%%%%%%%%%%%%%%%%%%%%%%%%
function [Gammaz1,Gammaz2,XI1,XI2]=fcn(q,q_dot,M1,L1,Me,de,I1,Lc1,Ie,Lce,Fd,g)
%#codegen
%Preallocate output
Y=zeros(2,9);
%Take apart the input
q1=q(1);
q2=-q(2);
q_dot1=q_dot(1);
q_dot2=-q_dot(2);
%
Gammaz=[(q_dot1+q_dot2) q_dot1*L1^2 (2*q_dot1+q_dot2)*L1*cos(q2) -(2*q_dot1+q_dot2)*L1*sin(q2);
    (q_dot1+q_dot2) 0 q_dot1*L1*cos(q2) -q_dot1*L1*sin(q2)];
Gammazdot=zeros(2,4);
XI=-[0 g*L1*cos(q1) g*cos(q1+q2) -g*sin(q1+q2); 
    0 0 (q_dot1+q_dot2)*q_dot1*L1*sin(q2) (q_dot1+q_dot2)*q_dot1*L1*cos(q2)];
Gammaz1=Gammaz(1,:);
Gammaz2=Gammaz(2,:);
XI1=XI(1,:);
XI2=XI(2,:);

== matlab function Controller/Adaptive Controller/Calculate W ==
  data: q input double; q_dot input double; Y1 output double; q_ddot input double; Y2 output double
%%%%%%%%%%%%%%%%%%%%%%%%%%%%%%%%%%%%%%%%%%%%%%%%%%%%%%%%%%%%%%%%%%%%%%%%%%%
% Daniel Wiese
% 2.152
% Robot Manipulator
%--------------------------------------------------------------------------
% Robot
%%%%%%%%%%%%%%%%%%%%%%%%%%%%%%%%%%%%%%%%%%%%%%%%%%%%%%%%%%%%%%%%%%%%%%%%%%%
function [Y1,Y2]=fcn(q,q_dot,q_ddot)
%#codegen
%Preallocate output
Y=zeros(2,9);
%Take apart the input
q1=q(1);
q2=q(2);
q_dot1=q_dot(1);
q_dot2=q_dot(2);
q_ddot1=q_ddot(1);
q_ddot2=q_ddot(2);
%Calculate the first row of Y
Y(1,1)=q_ddot1;
Y(1,2)=q_ddot2;
Y(1,3)=(2*q_ddot1+q_ddot2)*cos(q2)-(q_dot2*q_dot1+q_dot1*q_dot2+q_dot2*q_dot2)*sin(q2);
Y(1,4)=(2*q_ddot1+q_ddot2)*sin(q2)+(q_dot2*q_dot1+q_dot1*q_dot2+q_dot2*q_dot2)*cos(q2);
Y(1,5)=cos(q1);
Y(1,6)=cos(q1+q2);
Y(1,7)=-sin(q1+q2);
Y(1,8)=q_dot1;
Y(1,9)=0;
%Calculate the second row of Y
Y(2,1)=0;
Y(2,2)=q_ddot1+q_ddot2;
Y(2,3)=q_ddot1*cos(q2)+q_dot1*q_dot1*sin(q2);
Y(2,4)=q_ddot1*sin(q2)-q_dot1*q_dot1*cos(q2);
Y(2,5)=0;
Y(2,6)=cos(q1+q2);
Y(2,7)=-sin(q1+q2);
Y(2,8)=0;
Y(2,9)=q_dot2;
%each row
Y1=Y(1,:);
Y2=Y(2,:);
